simulink model "sampleModel1808"  (R2023a)
settings: Solver=VariableStepAuto  StartTime=0.0  StopTime=10.0  RelTol=1e-3
libraries: hdlsllib x4, simulink x3
settings Model: Creator=user1  LastModifiedBy=user1

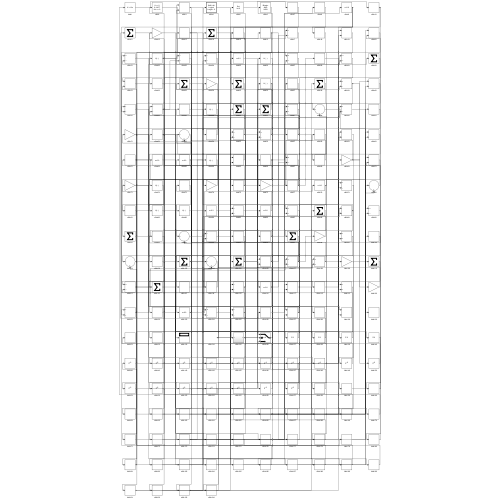
[thumbnail: Simulink's stored preview of the top-level diagram]
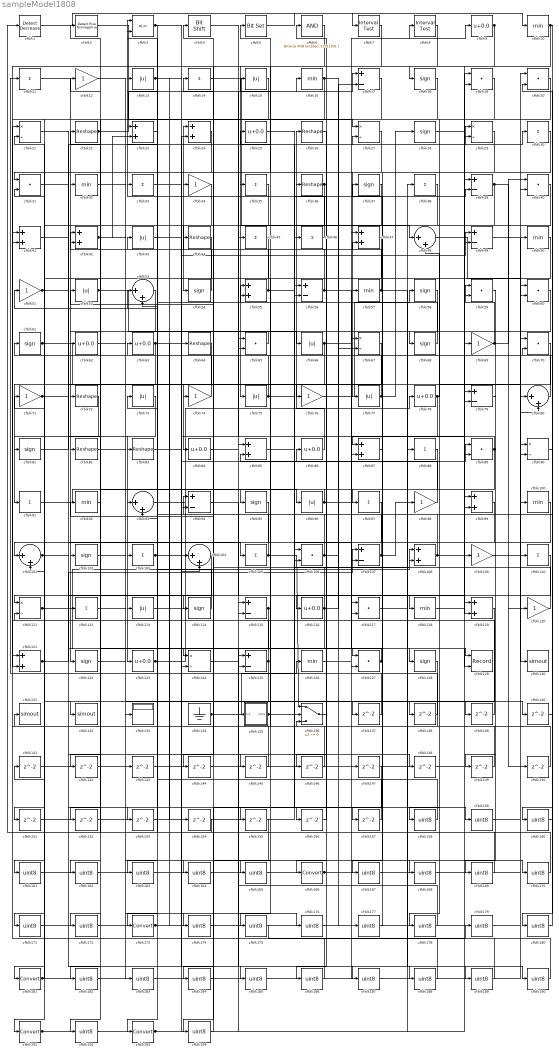
== system sampleModel1808 ==
  cfblk1 : simulink/Logic and Bit Operations/Detect Decrease  vinit=0.0  OutDataTypeStr=boolean
      settings: LibrarySourceBlock=|
      | hdlsllib/Logic and Bit
      | Operations/Detect
      | Decrease
  cfblk{10,16,32,50,57,92,100,118,126} (9 alike) : MinMax
  cfblk{48,53,80,93,101,104} (6 alike) : Sum  Inputs=|++
  cfblk{18,28,37,54,58,61,68,81,95,102,114,122,128} (13 alike) : Signum
  cfblk{11,14,30,33,35,38,45..46,88,91,97,103,105,110,112} (15 alike) : Sum  Inputs=+
  cfblk{19..20,31,40,59..60,65,70,89,106,117,127} (12 alike) : DotProduct  OutDataTypeStr=Inherit: Inherit via internal rule
  cfblk{17,39,49,56,79,94,107,115,125} (9 alike) : Sum  Inputs=+-
  cfblk{23..24,41..42,47,55,85,87,99,108,119,121} (12 alike) : Sum
  cfblk{12,34,51,69,71,74,76,98,109,120} (10 alike) : Gain
  cfblk{21,27,29,67,90,111,124} (7 alike) : Product  Inputs=*/  RndMeth=Zero  SaturateOnIntegerOverflow=on
  cfblk{13,15,43,52,66,73,75,77,96,113} (10 alike) : Abs  SaturateOnIntegerOverflow=off
  cfblk{9,25,62..63,78,84,86,116,123} (9 alike) : Bias  Bias=0.0  SaturateOnIntegerOverflow=off
  cfblk129 : Record  FileSettingsInternal="{\"entries\":[{\"content\":{\"excelSettings\":{\"content\":{},\"type\":\"Streamout.ExcelSettings\"}},\"type\":\"Streamout.FileSettingStorage\",\"uuid\":\"\"}],\"packageUris\":[\"http:\\/\\/schema.mathworks.com\\/mf0\\/streamout_blocks\\/R2020a\"],\"version\":\"1.0\"}"  Layout=[1 1]  SignalsInternal="{\"entries\":[{\"content\":{\"signals\":[{\"content\":{\"blockPath\":[],\"dimensions\":[1],\"domain\":\"\",\"lineColor\":\"#a2142f\",\"plots\":[1],\"port\":1,\"signalID\":4189,\"signalName\":\"XY Graph:1\"},\"type\":\"RecordBlkView.Signal\",\"uuid\":\"\"},{\"content\":{\"blockPath\":[],\"dimensions\":[1],\"domain\":\"\",\"lineColor\":\"#139fff\",\"plots\":[1],\"port\":2,\"signalID\":4192,\"signalName\":\"XY Graph:2\"},\"type\":\"RecordBlkView.Signal\",\"uuid\":\"\"}]},\"type\":\"RecordBlkView.InputSignals\",\"uuid\":\"\"}],\"packageUris\":[\"http:\\/\\/schema.mathworks.com\\/mf0\\/streamout_blocks\\/R2020a\"],\"version\":\"1.0\"}"  VisualizationBindings="{\"xyplotplugin\":{\"info\":[{\"series\":[{\"bindingParametersList\":[{\"parameter\":\"X-Axis\",\"signalID\":4189,\"signalName\":\"XY Graph:1\"},{\"parameter\":\"Y-Axis\",\"signalID\":4192,\"signalName\":\"XY Graph:2\"}],\"seriesID\":31353}],\"subplotID\":1}]}}"  CompatibilityTag=XY  st=-1
  cfblk130 : ToWorkspace  VariableName=simout  SaveFormat=Timeseries  SampleTime=-1
  cfblk131 : ToWorkspace  VariableName=simout  SaveFormat=Timeseries  SampleTime=-1
  cfblk132 : ToWorkspace  VariableName=simout  SaveFormat=Timeseries  SampleTime=-1
  cfblk133 : Display
  cfblk134 : Ground
  cfblk135 : Subsystem
      settings: LibrarySourceBlock=|
      | hdlsllib/Ports &
      | Subsystems/Subsystem
  cfblk136 : Switch  SaturateOnIntegerOverflow=off  InputSameDT=off
  cfblk{137..157} (21 alike) : Delay  SampleTime=1
  cfblk{158..165,167..172,174..180,182..190,192,194} (32 alike) : DataTypeConversion  OutDataTypeStr=uint8  SaturateOnIntegerOverflow=off  RndMeth=Floor
  cfblk{166,173,181,191,193} (5 alike) : DataTypeConversion  SaturateOnIntegerOverflow=off  RndMeth=Floor
  cfblk2 : hdlsllib/Logic and Bit Operations/Detect Rise Nonnegative  vinit=0  OutDataTypeStr=boolean
  cfblk{22,26,36,44,64,72,82..83} (8 alike) : Reshape
  cfblk3 : RelationalOperator  Operator=<=  OutDataTypeStr=boolean  InputSameDT=off
  cfblk4 : hdlsllib/Logic and Bit Operations/Bit Shift  mode=Shift Left Logical  N=0
  cfblk5 : simulink/Logic and Bit Operations/Bit Set  iBit=0
      settings: LibrarySourceBlock=|
      | hdlsllib/Logic and Bit
      | Operations/Bit Set
  cfblk6 : simulink/Logic and Bit Operations/Bitwise Operator  logicop=AND  UseBitMask=on  BitMask=bin2dec('11011001')  BitMaskRealWorld=Stored Integer
      settings: LibrarySourceBlock=|
      | hdlsllib/Logic and Bit
      | Operations/Bitwise
      | Operator
  cfblk7 : hdlsllib/Logic and Bit Operations/Interval Test  IntervalClosedRight=on  uplimit=0.5  IntervalClosedLeft=on  lowlimit=-0.5  OutDataTypeStr=boolean
  cfblk8 : hdlsllib/Logic and Bit Operations/Interval Test  IntervalClosedRight=on  uplimit=0.5  IntervalClosedLeft=on  lowlimit=-0.5  OutDataTypeStr=boolean
  wires:
  cfblk17/1 -> cfblk122/1
  cfblk86/1 -> cfblk26/1
  cfblk90/1 -> cfblk63/1
  cfblk136/1 -> cfblk6/1
  cfblk11/1 -> cfblk32/1
  cfblk57/1 -> cfblk24/1, cfblk190/1
  cfblk42/1 -> cfblk23/2, cfblk174/1
  cfblk116/1 -> cfblk52/1, cfblk67/2, cfblk165/1
  cfblk46/1 -> cfblk3/1
  cfblk76/1 -> cfblk58/1
  cfblk77/1 -> cfblk42/1, cfblk28/1, cfblk55/2
  cfblk6/1 -> cfblk75/1
  cfblk37/1 -> cfblk54/1
  cfblk67/1 -> cfblk91/1
  cfblk104/1 -> cfblk181/1
  cfblk39/1 -> cfblk68/1, cfblk120/1
  cfblk105/1 -> cfblk136/1, cfblk29/1, cfblk43/1
  cfblk50/1 -> cfblk173/1
  cfblk63/1 -> cfblk102/1, cfblk129/2
  cfblk115/1 -> cfblk11/1, cfblk55/1
  cfblk89/1 -> cfblk87/1, cfblk112/1
  cfblk15/1 -> cfblk72/1
  cfblk54/1 -> cfblk44/1
  cfblk45/1 -> cfblk191/1
  cfblk69/1 -> cfblk59/1, cfblk40/1, cfblk150/1
  cfblk18/1 -> cfblk81/1
  cfblk73/1 -> cfblk123/1
  cfblk34/1 -> cfblk193/1
  cfblk123/1 -> cfblk78/1, cfblk23/1
  cfblk100/1 -> cfblk166/1
  cfblk68/1 -> cfblk33/1
  cfblk106/1 -> cfblk17/2, cfblk51/1, cfblk146/1
  cfblk24/1 -> cfblk31/1
  cfblk48/1 -> cfblk130/1
  cfblk80/1 -> cfblk5/1
  cfblk2/1 -> cfblk27/1
  cfblk125/1 -> cfblk111/2, cfblk162/1
  cfblk14/1 -> cfblk48/1
  cfblk52/1 -> cfblk66/1, cfblk156/1
  cfblk134/1 -> cfblk126/1, cfblk94/1, cfblk17/1
  cfblk1/1 -> cfblk10/1
  cfblk72/1 -> cfblk101/1
  cfblk101/1 -> cfblk31/2, cfblk145/1
  cfblk49/1 -> cfblk90/1
  cfblk16/1 -> cfblk82/1, cfblk151/1, cfblk177/1
  cfblk64/1 -> cfblk84/1
  cfblk27/1 -> cfblk77/1
  cfblk88/1 -> cfblk97/1
  cfblk19/1 -> cfblk41/2
  cfblk108/1 -> cfblk25/1, cfblk30/1
  cfblk9/1 -> cfblk121/2, cfblk74/1, cfblk93/2
  cfblk96/1 -> cfblk95/1, cfblk9/1
  cfblk92/1 -> cfblk132/1
  cfblk71/1 -> cfblk105/1, cfblk153/1
  cfblk121/1 -> cfblk101/2, cfblk107/1
  cfblk61/1 -> cfblk80/2, cfblk125/2
  cfblk74/1 -> cfblk61/1
  cfblk65/1 -> cfblk62/1
  cfblk103/1 -> cfblk89/1, cfblk49/2
  cfblk22/1 -> cfblk16/1, cfblk137/1
  cfblk87/1 -> cfblk127/1
  cfblk81/1 -> cfblk27/2
  cfblk66/1 -> cfblk29/2, cfblk172/1
  cfblk113/1 -> cfblk56/1
  cfblk91/1 -> cfblk96/1
  cfblk41/1 -> cfblk114/1
  cfblk4/1 -> cfblk89/2
  cfblk5/1 -> cfblk7/1
  cfblk109/1 -> cfblk90/2
  cfblk58/1 -> cfblk67/1
  cfblk94/1 -> cfblk118/1
  cfblk3/1 -> cfblk103/1, cfblk140/1
  cfblk78/1 -> cfblk48/2, cfblk157/1
  cfblk127/1 -> cfblk124/1, cfblk37/1
  cfblk118/1 -> cfblk79/1
  cfblk114/1 -> cfblk13/1
  cfblk120/1 -> cfblk92/1
  cfblk7/1 -> cfblk35/1
  cfblk85/1 -> cfblk39/2
  cfblk128/1 -> cfblk131/1
  cfblk10/1 -> cfblk99/2, cfblk160/1
  cfblk28/1 -> cfblk119/1
  cfblk111/1 -> cfblk108/1, cfblk133/1
  cfblk126/1 -> cfblk8/1
  cfblk51/1 -> cfblk83/1, cfblk79/2
  cfblk55/1 -> cfblk3/2, cfblk159/1
  cfblk43/1 -> cfblk87/2
  cfblk93/1 -> cfblk46/1
  cfblk40/1 -> cfblk57/1
  cfblk25/1 -> cfblk129/1
  cfblk75/1 -> cfblk22/1, cfblk107/2
  cfblk8/1 -> cfblk18/1
  cfblk26/1 -> cfblk76/1
  cfblk98/1 -> cfblk15/1
  cfblk33/1 -> cfblk119/2
  cfblk31/1 -> cfblk124/2
  cfblk99/1 -> cfblk113/1
  cfblk84/1 -> cfblk49/1
  cfblk56/1 -> cfblk128/1, cfblk2/1
  cfblk23/1 -> cfblk93/1
  cfblk107/1 -> cfblk4/1, cfblk98/1, cfblk14/1
  cfblk135/1(Out1) -> cfblk106/1, cfblk108/2
  cfblk36/1 -> cfblk116/1, cfblk106/2
  cfblk95/1 -> cfblk111/1
  cfblk13/1 -> cfblk154/1, cfblk187/1
  cfblk137/1 -> cfblk42/2
  cfblk82/1 -> cfblk138/1
  cfblk138/1 -> cfblk53/2
  cfblk102/1 -> cfblk139/1
  cfblk139/1 -> cfblk41/1
  cfblk141/1 -> cfblk19/1
  cfblk44/1 -> cfblk142/1
  cfblk112/1 -> cfblk143/1
  cfblk143/1 -> cfblk39/1
  cfblk35/1 -> cfblk144/1
  cfblk144/1 -> cfblk115/2
  cfblk145/1 -> cfblk121/1
  cfblk146/1 -> cfblk85/2
  cfblk83/1 -> cfblk148/1
  cfblk148/1 -> cfblk99/1
  cfblk59/1 -> cfblk149/1
  cfblk149/1 -> cfblk125/1
  cfblk150/1 -> cfblk136/3
  cfblk151/1 -> cfblk136/2
  cfblk29/1 -> cfblk152/1
  cfblk153/1 -> cfblk56/2
  cfblk154/1 -> cfblk1/1
  cfblk97/1 -> cfblk155/1
  cfblk156/1 -> cfblk36/1
  cfblk157/1 -> cfblk73/1
  cfblk70/1 -> cfblk158/1
  cfblk158/1 -> cfblk86/1
  cfblk159/1 -> cfblk70/1
  cfblk160/1 -> cfblk70/2
  cfblk38/1 -> cfblk161/1
  cfblk161/1 -> cfblk135/1(In1)
  cfblk162/1 -> cfblk38/1
  cfblk60/1 -> cfblk163/1
  cfblk163/1 -> cfblk109/1
  cfblk32/1 -> cfblk164/1
  cfblk164/1 -> cfblk60/1
  cfblk165/1 -> cfblk60/2
  cfblk166/1 -> cfblk127/2, cfblk80/1
  cfblk30/1 -> cfblk167/1
  cfblk167/1 -> cfblk100/1
  cfblk12/1 -> cfblk168/1
  cfblk168/1 -> cfblk69/1
  cfblk79/1 -> cfblk169/1
  cfblk169/1 -> cfblk12/1
  cfblk117/1 -> cfblk170/1
  cfblk170/1 -> cfblk53/1
  cfblk119/1 -> cfblk171/1
  cfblk171/1 -> cfblk117/1
  cfblk172/1 -> cfblk117/2
  cfblk173/1 -> cfblk59/2, cfblk64/1, cfblk85/1
  cfblk174/1 -> cfblk50/1
  cfblk47/1 -> cfblk175/1
  cfblk142/1 -> cfblk176/1
  cfblk176/1 -> cfblk47/1
  cfblk177/1 -> cfblk47/2
  cfblk20/1 -> cfblk178/1
  cfblk178/1 -> cfblk115/1
  cfblk175/1 -> cfblk179/1
  cfblk179/1 -> cfblk20/1
  cfblk140/1 -> cfblk180/1
  cfblk180/1 -> cfblk20/2
  cfblk181/1 -> cfblk40/2, cfblk71/1
  cfblk152/1 -> cfblk182/1
  cfblk182/1 -> cfblk104/1
  cfblk62/1 -> cfblk183/1
  cfblk183/1 -> cfblk104/2
  cfblk147/1 -> cfblk184/1
  cfblk184/1 -> cfblk65/2
  cfblk122/1 -> cfblk185/1
  cfblk185/1 -> cfblk147/1
  cfblk110/1 -> cfblk186/1
  cfblk186/1 -> cfblk65/1
  cfblk187/1 -> cfblk110/1
  cfblk21/1 -> cfblk188/1
  cfblk188/1 -> cfblk141/1
  cfblk124/1 -> cfblk189/1
  cfblk189/1 -> cfblk21/1
  cfblk190/1 -> cfblk21/2
  cfblk191/1 -> cfblk94/2, cfblk19/2
  cfblk53/1 -> cfblk192/1
  cfblk192/1 -> cfblk45/1
  cfblk193/1 -> cfblk24/2, cfblk88/1
  cfblk155/1 -> cfblk194/1
  cfblk194/1 -> cfblk34/1

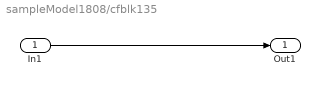
== system sampleModel1808/cfblk135 ==
  In1 : Inport
  Out1 : Outport
  wires:
  In1/1 -> Out1/1
